simulink model "Q9_Q10_Q11_statespace"  (R2022a)
settings: Solver=VariableStepAuto  StartTime=0.0  StopTime=5  RelTol=1e-3
undefined symbols (not defined in the file): C, E, Ge, H, K, k_follow, L, Ts
settings Model: Creator=Asus  LastModifiedBy=fatae
settings SolverCC: AlgebraicLoopSolver=TrustRegion
settings DataIOCC: ReturnWorkspaceOutputs=off
settings DebuggingCC: UnconnectedInputMsg=warning  UnconnectedOutputMsg=warning  UnconnectedLineMsg=warning  SFMachineParentedDataDiag=warning  ArithmeticOperatorsInVariantConditions=warning
settings SFSimCC: CustomCodeUndefinedFunction=UseInterfaceOnly

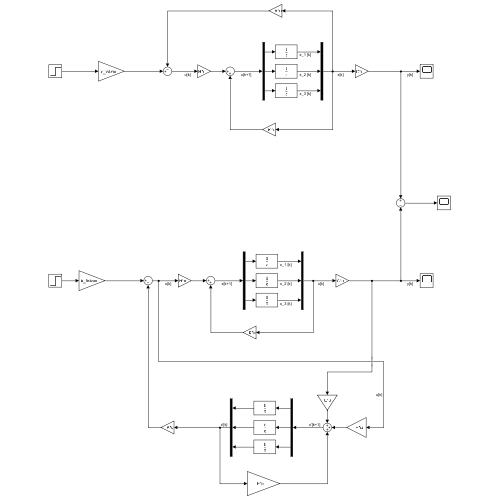
[thumbnail: Simulink's stored preview of the top-level diagram]
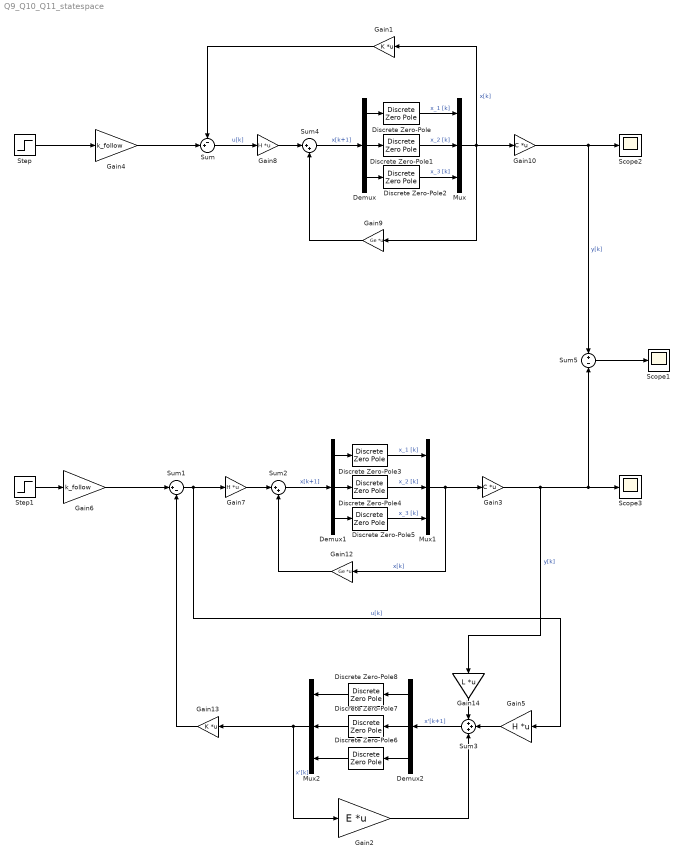
== system Q9_Q10_Q11_statespace ==
  Demux : Demux  Outputs=3
  Demux1 : Demux  Outputs=3
  Demux2 : Demux  Outputs=3
  Discrete Zero-Pole{,1..8} (9 alike) : DiscreteZeroPole  Zeros=[]  Poles=[0]  Gain=1  SampleTime=Ts(2)
  Gain1 : Gain  Gain=K  Multiplication=Matrix(K*u)
  Gain10 : Gain  Gain=C  Multiplication=Matrix(K*u)
  Gain12 : Gain  Gain=Ge  Multiplication=Matrix(K*u)
  Gain13 : Gain  Gain=K  Multiplication=Matrix(K*u)
  Gain14 : Gain  Gain=L  Multiplication=Matrix(K*u)
  Gain2 : Gain  Gain=E  Multiplication=Matrix(K*u)
  Gain3 : Gain  Gain=C  Multiplication=Matrix(K*u)
  Gain4 : Gain  Gain=k_follow
  Gain5 : Gain  Gain=H  Multiplication=Matrix(K*u)
  Gain6 : Gain  Gain=k_follow
  Gain7 : Gain  Gain=H  Multiplication=Matrix(K*u)
  Gain8 : Gain  Gain=H  Multiplication=Matrix(K*u)
  Gain9 : Gain  Gain=Ge  Multiplication=Matrix(K*u)
  Mux : Mux  Inputs=3
  Mux1 : Mux  Inputs=3
  Mux2 : Mux  Inputs=3
  Scope1 : Scope
  Scope2 : Scope
  Scope3 : Scope
  Step : Step  Time=0  SampleTime=0
  Step1 : Step  Time=0  SampleTime=0
  Sum : Sum  Inputs=-+|
  Sum1 : Sum  Inputs=|+-
  Sum2 : Sum  Inputs=|++
  Sum3 : Sum  Inputs=+++
  Sum4 : Sum  Inputs=|++
  Sum5 : Sum  Inputs=+|-
  wires:
  Gain8/1 -> Sum4/1
  Discrete Zero-Pole/1 -> Mux/1  "x_1 [k]"
  Gain10/1 -> Scope2/1, Sum5/1  "y[k]"
  Gain9/1 -> Sum4/2
  Sum4/1 -> Demux/1  "x[k+1]"
  Demux/1 -> Discrete Zero-Pole/1
  Demux/2 -> Discrete Zero-Pole1/1
  Demux/3 -> Discrete Zero-Pole2/1
  Mux/1 -> Gain9/1, Gain10/1, Gain1/1  "x[k]"
  Discrete Zero-Pole1/1 -> Mux/2  "x_2 [k]"
  Discrete Zero-Pole2/1 -> Mux/3  "x_3 [k]"
  Sum/1 -> Gain8/1  "u[k]"
  Gain1/1 -> Sum/1
  Gain4/1 -> Sum/2
  Step/1 -> Gain4/1
  Step1/1 -> Gain6/1
  Gain6/1 -> Sum1/1
  Mux1/1 -> Gain12/1, Gain3/1  "x[k]"
  Sum2/1 -> Demux1/1  "x[k+1]"
  Demux1/2 -> Discrete Zero-Pole4/1
  Sum1/1 -> Gain5/1, Gain7/1  "u[k]"
  Discrete Zero-Pole4/1 -> Mux1/2  "x_2 [k]"
  Demux1/1 -> Discrete Zero-Pole3/1
  Gain12/1 -> Sum2/2
  Discrete Zero-Pole3/1 -> Mux1/1  "x_1 [k]"
  Gain3/1 -> Gain14/1, Sum5/2, Scope3/1  "y[k]"
  Discrete Zero-Pole5/1 -> Mux1/3  "x_3 [k]"
  Demux1/3 -> Discrete Zero-Pole5/1
  Gain7/1 -> Sum2/1
  Demux2/1 -> Discrete Zero-Pole8/1
  Demux2/2 -> Discrete Zero-Pole7/1
  Demux2/3 -> Discrete Zero-Pole6/1
  Discrete Zero-Pole8/1 -> Mux2/1
  Discrete Zero-Pole7/1 -> Mux2/2
  Discrete Zero-Pole6/1 -> Mux2/3
  Mux2/1 -> Gain13/1, Gain2/1  "x'[k]"
  Sum3/1 -> Demux2/1  "x'[k+1]"
  Gain2/1 -> Sum3/3
  Gain5/1 -> Sum3/2
  Gain14/1 -> Sum3/1
  Gain13/1 -> Sum1/2
  Sum5/1 -> Scope1/1
